simulink model "TempCorrect_OfflineTest_del"  (R2014a)
settings: Solver=ode3  StartTime=0.0  StopTime=Gyro.time(end)  FixedStep=1/400  RelTol=1e-3
settings Model: ExtModeTrigDuration=40001  Creator=darenlee  LastModifiedBy=darenlee
settings DataIOCC: SignalLoggingSaveFormat=ModelDataLogs
settings DebuggingCC: MultiTaskDSMMsg=warning  MultiTaskCondExecSysMsg=none
settings RTWCC: IncludeERTFirstTime=on

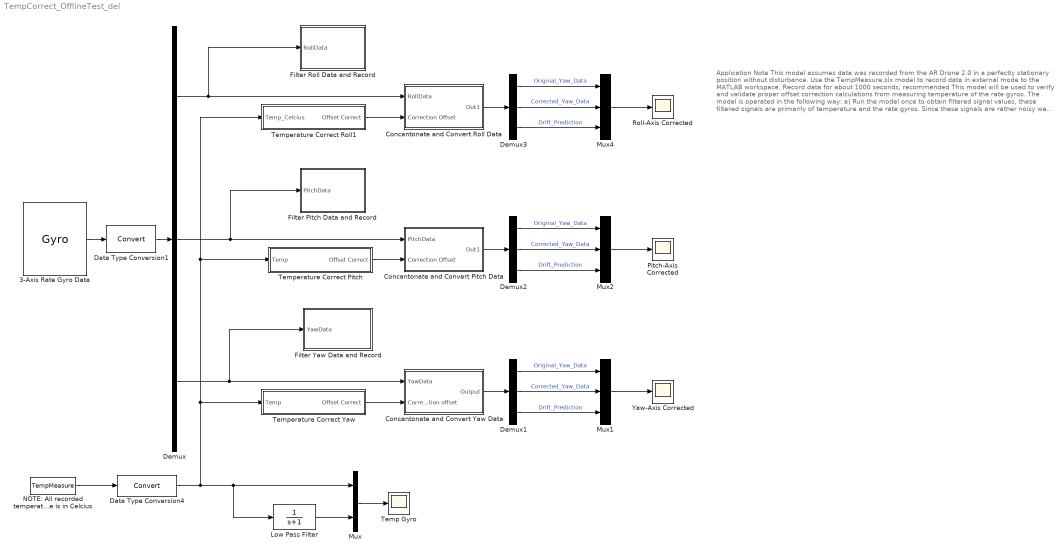
== system TempCorrect_OfflineTest_del ==
  note: Application Note
      |
      | This model assumes data was recorded from the AR Drone 2.0 in a perfectly stationary position without disturbance. Use the TempMeasure.slx model to record data in external mode to the MATLAB workspace. Record data for about 1000 seconds, recommended
      |
      | This model will be used to verify and validate proper
      | offset correction calculations from measuring temperature of the rate gyros. The model is operated
      | in the following way:
      |
      | a)
      | Run the model once to obtain filtered signal values, these filtered signals are primarily of temperature and the rate gyros. Since these signals are rather noisy we want to be able to find the average value of these signals to get a better estimate of the offset parameters
      |
      | b)
      | Run the script 'Curve_Fit.m' one cell at a time . The first cell will find the linear parameters for roll, the second cell for pitch and the third cell for yaw.
      | The curve fit will be between two workspace variables, as an example
      |
      | 'TempMeasureRefined' which is the indepdent 'x' variable
      | 'GyroDrift_Roll' which is the dependent 'y' variable
      |
      | and so forth
      |
      | Do a linear polymoial y=ax+b fit and make note of what the equation is. Update the following subsytems in this model with the parameters found in the curve fit
      |
      | \Temperature Correct Roll
      | \Temperature Correct Pitch
      | \Temperature Correct Yaw
      |
      | c)
      | Now, we'r eready to validate. Press the play button and look at the scopes.
      | Yellow Signal - The original uncorrected data not centered at zero
      | Purple Signal - Corrected data. This should be centered at zero
      | Teal Signal - The purpose of this is to examine integration drift.. it is a measurement of how effective our correction factor removed the drift bias. If one were to integrate the purple signal, ideally the reported attitude should be zero or close to it. Minor drift is acceptable since the AHRS system will take care of the rest
  3-Axis Rate Gyro Data : FromWorkspace  VariableName=Gyro
  Concantonate and Convert Pitch Data : Subsystem
  Concantonate and Convert Roll Data : Subsystem
  Concantonate and Convert Yaw Data : Subsystem
  Data Type Conversion1 : DataTypeConversion
  Data Type Conversion4 : DataTypeConversion
  Demux{,1..3} (4 alike) : Demux  Outputs=3
  Filter Pitch Data and Record : Subsystem
  Filter Roll Data and Record : Subsystem
  Filter Yaw Data and Record : Subsystem
  Low Pass Filter : TransferFcn  Denominator=[1 1]
  Mux : Mux  Inputs=2
  Mux1 : Mux  Inputs=3
  Mux2 : Mux  Inputs=3
  Mux4 : Mux  Inputs=3
  NOTE: All recorded temperature is in Celcius : FromWorkspace  VariableName=TempMeasure
  Pitch-Axis Corrected : Scope
      settings: YMin=-50  YMax=1000  SaveName=Pitch_Corrected_Uncorrected
  Roll-Axis Corrected : Scope
      settings: TimeRange=571.1351351351351  YMin=-40  SaveName=Roll_Corrected_Uncorrected
  Temp Gyro : Scope
      settings: YMin=0  YMax=55000  SaveName=FilteredTemp
  Temperature Correct Pitch : Subsystem
  Temperature Correct Roll1 : Subsystem
  Temperature Correct Yaw : Subsystem
  Yaw-Axis Corrected : Scope
      settings: ShowLegends=on  YMin=-12  SaveName=Roll_Corrected_Uncorrected2
  wires:
  3-Axis Rate Gyro Data/1 -> Data Type Conversion1/1
  NOTE: All recorded temperature is in Celcius/1 -> Data Type Conversion4/1
  Data Type Conversion1/1 -> Demux/1
  Demux/1 -> Concantonate and Convert Roll Data/1(RollData), Filter Roll Data and Record/1(RollData)
  Data Type Conversion4/1 -> Mux/1, Low Pass Filter/1, Temperature Correct Roll1/1(Temp_Celcius), Temperature Correct Pitch/1(Temp), Temperature Correct Yaw/1(Temp)
  Mux/1 -> Temp Gyro/1
  Demux/3 -> Concantonate and Convert Yaw Data/1(YawData), Filter Yaw Data and Record/1(YawData)
  Low Pass Filter/1 -> Mux/2
  Demux/2 -> Concantonate and Convert Pitch Data/1(PitchData), Filter Pitch Data and Record/1(PitchData)
  Temperature Correct Yaw/1(Offset Correct) -> Concantonate and Convert Yaw Data/2(Correction offset)
  Concantonate and Convert Yaw Data/1(Output) -> Demux1/1
  Demux1/1 -> Mux1/1  "Original_Yaw_Data"
  Demux1/2 -> Mux1/2  "Corrected_Yaw_Data"
  Demux1/3 -> Mux1/3  "Drift_Prediction"
  Mux1/1 -> Yaw-Axis Corrected/1
  Temperature Correct Pitch/1(Offset Correct) -> Concantonate and Convert Pitch Data/2(Correction Offset)
  Concantonate and Convert Pitch Data/1(Out1) -> Demux2/1
  Demux2/1 -> Mux2/1  "Original_Yaw_Data"
  Demux2/2 -> Mux2/2  "Corrected_Yaw_Data"
  Demux2/3 -> Mux2/3  "Drift_Prediction"
  Mux2/1 -> Pitch-Axis Corrected/1
  Temperature Correct Roll1/1(Offset Correct) -> Concantonate and Convert Roll Data/2(Correction Offset)
  Demux3/1 -> Mux4/1  "Original_Yaw_Data"
  Demux3/2 -> Mux4/2  "Corrected_Yaw_Data"
  Demux3/3 -> Mux4/3  "Drift_Prediction"
  Concantonate and Convert Roll Data/1(Out1) -> Demux3/1
  Mux4/1 -> Roll-Axis Corrected/1

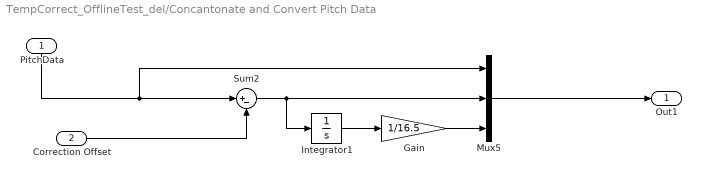
== system TempCorrect_OfflineTest_del/Concantonate and Convert Pitch Data ==
  PitchData : Inport
  Correction Offset : Inport  Port=2
  Gain : Gain  Gain=1/16.5
  Integrator1 : Integrator
  Mux5 : Mux  Inputs=3
  Sum2 : Sum  Inputs=|+-
  Out1 : Outport
  wires:
  Mux5/1 -> Out1/1
  Sum2/1 -> Integrator1/1, Mux5/2
  Correction Offset/1 -> Sum2/2
  Gain/1 -> Mux5/3
  Integrator1/1 -> Gain/1
  PitchData/1 -> Mux5/1, Sum2/1

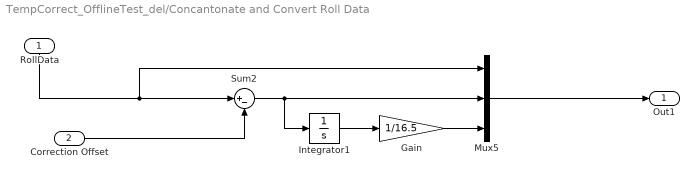
== system TempCorrect_OfflineTest_del/Concantonate and Convert Roll Data ==
  RollData : Inport
  Correction Offset : Inport  Port=2
  Gain : Gain  Gain=1/16.5
  Integrator1 : Integrator
  Mux5 : Mux  Inputs=3
  Sum2 : Sum  Inputs=|+-
  Out1 : Outport
  wires:
  Mux5/1 -> Out1/1
  Sum2/1 -> Integrator1/1, Mux5/2
  Correction Offset/1 -> Sum2/2
  Gain/1 -> Mux5/3
  Integrator1/1 -> Gain/1
  RollData/1 -> Mux5/1, Sum2/1

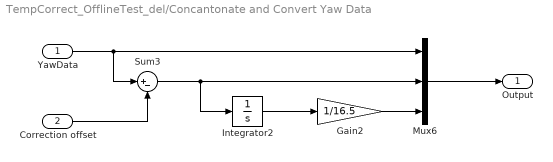
== system TempCorrect_OfflineTest_del/Concantonate and Convert Yaw Data ==
  YawData : Inport
  Correction offset : Inport  Port=2
  Gain2 : Gain  Gain=1/16.5
  Integrator2 : Integrator
  Mux6 : Mux  Inputs=3
  Sum3 : Sum  Inputs=|+-
  Output : Outport
  wires:
  Sum3/1 -> Integrator2/1, Mux6/2
  Correction offset/1 -> Sum3/2
  Integrator2/1 -> Gain2/1
  Mux6/1 -> Output/1
  Gain2/1 -> Mux6/3
  YawData/1 -> Sum3/1, Mux6/1

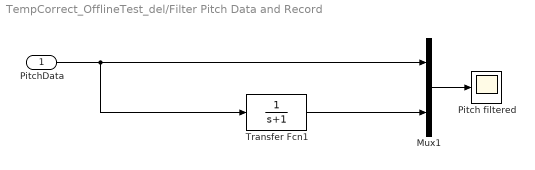
== system TempCorrect_OfflineTest_del/Filter Pitch Data and Record ==
  PitchData : Inport
  Mux1 : Mux  Inputs=2
  Pitch filtered : Scope
      settings: SaveName=Pitch_Gyro_filtered
  Transfer Fcn1 : TransferFcn  Denominator=[1 1]
  wires:
  Transfer Fcn1/1 -> Mux1/2
  Mux1/1 -> Pitch filtered/1
  PitchData/1 -> Transfer Fcn1/1, Mux1/1

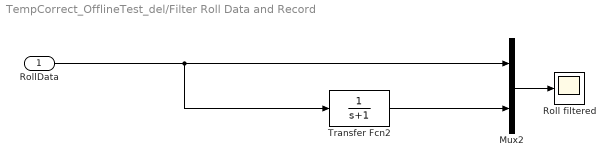
== system TempCorrect_OfflineTest_del/Filter Roll Data and Record ==
  RollData : Inport
  Mux2 : Mux  Inputs=2
  Roll filtered : Scope
      settings: SaveName=Roll_Gyro_filtered
  Transfer Fcn2 : TransferFcn  Denominator=[1 1]
  wires:
  Mux2/1 -> Roll filtered/1
  Transfer Fcn2/1 -> Mux2/2
  RollData/1 -> Transfer Fcn2/1, Mux2/1

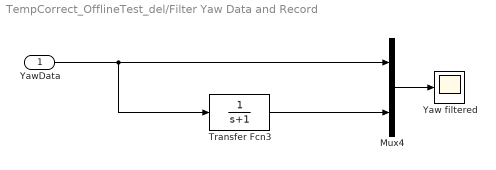
== system TempCorrect_OfflineTest_del/Filter Yaw Data and Record ==
  YawData : Inport
  Mux4 : Mux  Inputs=2
  Transfer Fcn3 : TransferFcn  Denominator=[1 1]
  Yaw filtered : Scope
      settings: SaveName=Yaw_Gyro_filtered
  wires:
  Mux4/1 -> Yaw filtered/1
  Transfer Fcn3/1 -> Mux4/2
  YawData/1 -> Transfer Fcn3/1, Mux4/1

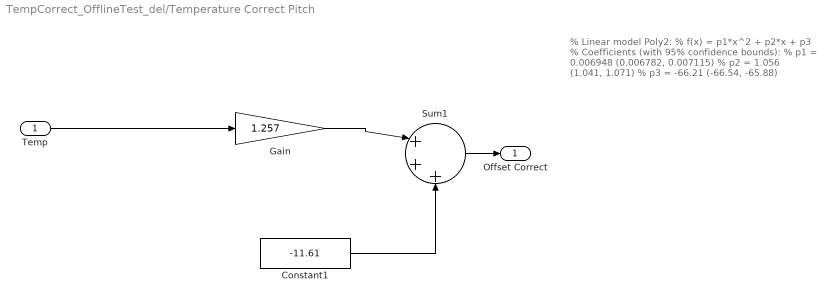
== system TempCorrect_OfflineTest_del/Temperature Correct Pitch ==
  note: % Linear model Poly2:
      | %      f(x) = p1*x^2 + p2*x + p3
      | % Coefficients (with 95% confidence bounds):
      | %        p1 =    0.006948  (0.006782, 0.007115)
      | %        p2 =       1.056  (1.041, 1.071)
      | %        p3 =      -66.21  (-66.54, -65.88)
  Temp : Inport
  Constant1 : Constant  Value=-11.61
  Gain : Gain  Gain=1.257
  Sum1 : Sum  Inputs=|+++
  Offset Correct : Outport
  wires:
  Temp/1 -> Gain/1
  Constant1/1 -> Sum1/3
  Sum1/1 -> Offset Correct/1
  Gain/1 -> Sum1/1

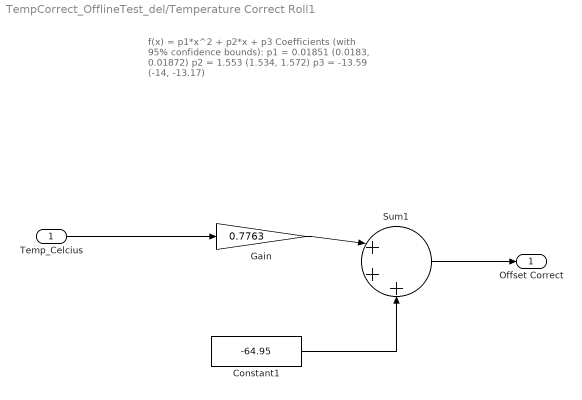
== system TempCorrect_OfflineTest_del/Temperature Correct Roll1 ==
  note: f(x) = p1*x^2 + p2*x + p3
      | Coefficients (with 95% confidence bounds):
      |        p1 =     0.01851  (0.0183, 0.01872)
      |        p2 =       1.553  (1.534, 1.572)
      |        p3 =      -13.59  (-14, -13.17)
  Temp_Celcius : Inport
  Constant1 : Constant  Value=-64.95
  Gain : Gain  Gain=0.7763
  Sum1 : Sum  Inputs=|+++
  Offset Correct : Outport
  wires:
  Temp_Celcius/1 -> Gain/1
  Gain/1 -> Sum1/1
  Constant1/1 -> Sum1/3
  Sum1/1 -> Offset Correct/1

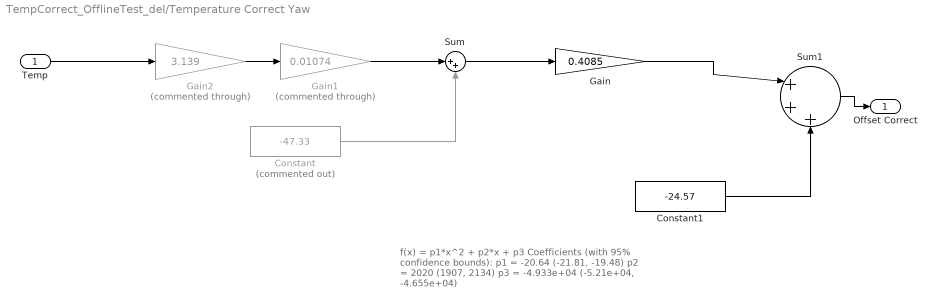
== system TempCorrect_OfflineTest_del/Temperature Correct Yaw ==
  note: f(x) = p1*x^2 + p2*x + p3
      | Coefficients (with 95% confidence bounds):
      |        p1 =      -20.64  (-21.81, -19.48)
      |        p2 =        2020  (1907, 2134)
      |        p3 =  -4.933e+04  (-5.21e+04, -4.655e+04)
  Temp : Inport
  Constant : Constant  Commented=on  Value=-47.33
  Constant1 : Constant  Value=-24.57
  Gain : Gain  Gain=0.4085
  Gain1 : Gain  Commented=through  Gain=0.01074
  Gain2 : Gain  Commented=through  Gain=3.139
  Sum : Sum  Inputs=|++
  Sum1 : Sum  Inputs=|+++
  Offset Correct : Outport
  wires:
  Sum1/1 -> Offset Correct/1
  Constant1/1 -> Sum1/3
  Gain/1 -> Sum1/1
  Sum/1 -> Gain/1
  Temp/1 -> Gain2/1
  Gain1/1 -> Sum/1
  Constant/1 -> Sum/2
  Gain2/1 -> Gain1/1
